simulink subsystem "galvo_cao"  (R2021a)
settings: Solver=VariableStepAuto  StartTime=0.0  StopTime=10.0  RelTol=1e-3
settings Model: Creator=billy  LastModifiedBy=billy

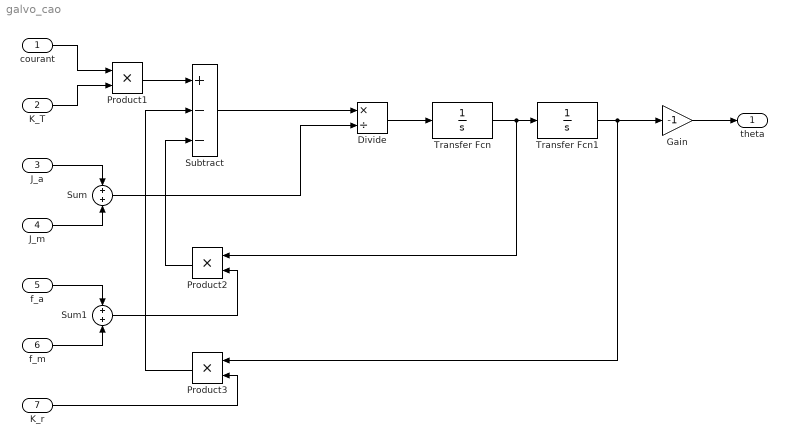
== system galvo_cao ==
  courant : Inport
  K_T : Inport  Port=2
  J_a : Inport  Port=3
  J_m : Inport  Port=4
  f_a : Inport  Port=5
  f_m : Inport  Port=6
  K_r : Inport  Port=7
  Divide : Product  Inputs=*/
  Gain : Gain  Gain=-1
  Product1 : Product
  Product2 : Product
  Product3 : Product
  Subtract : Sum  Inputs=+--
  Sum : Sum  Inputs=+|+
  Sum1 : Sum  Inputs=+|+
  Transfer Fcn : TransferFcn  Denominator=[1 0]
  Transfer Fcn1 : TransferFcn  Denominator=[1 0]
  theta : Outport
  wires:
  J_a/1 -> Sum/1
  J_m/1 -> Sum/2
  Sum/1 -> Divide/2
  Subtract/1 -> Divide/1
  Product1/1 -> Subtract/1
  Divide/1 -> Transfer Fcn/1
  f_m/1 -> Sum1/2
  f_a/1 -> Sum1/1
  Sum1/1 -> Product2/2
  Transfer Fcn/1 -> Transfer Fcn1/1, Product2/1
  Product2/1 -> Subtract/3
  Transfer Fcn1/1 -> Product3/1, Gain/1
  K_r/1 -> Product3/2
  Product3/1 -> Subtract/2
  courant/1 -> Product1/1
  K_T/1 -> Product1/2
  Gain/1 -> theta/1
